simulink model "untitled"  (R2018a)
settings: Solver=VariableStepAuto  StartTime=0.0  StopTime=10.0  RelTol=1e-3
settings Model: Creator=fredd  LastModifiedBy=fredd

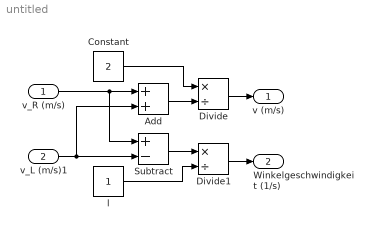
== system untitled ==
  v_R (m/s) : Inport
  v_L (m/s)1 : Inport  Port=2
  Add : Sum
  Constant : Constant  Value=2
  Divide : Product  Inputs=*/
  Divide1 : Product  Inputs=*/
  Subtract : Sum  Inputs=+-
  l : Constant
  v (m/s) : Outport
  " Winkelgeschwindigkeit (1/s)" : Outport  Port=2
  wires:
  v_R (m/s)/1 -> Subtract/1, Add/1
  v_L (m/s)1/1 -> Subtract/2, Add/2
  Add/1 -> Divide/2
  Constant/1 -> Divide/1
  Divide/1 -> v (m/s)/1
  Subtract/1 -> Divide1/1
  l/1 -> Divide1/2
  Divide1/1 -> " Winkelgeschwindigkeit (1/s)"/1
